simulink model "DynamicalMediationModel_Sim"  (R2015a)
settings: Solver=ode45  StartTime=0.0  StopTime=36  RelTol=1e-3
values from neighbouring files (symbols this model uses):
  out_model = pem(out_iddata',[pC_struct pB_struct])    [DynamicalModelingExercise_code.m]
  StepTime = 8    [DynamicalModelingExercise_code.m]
libraries: slident x3
settings Model: Creator=ktimms  LastModifiedBy=timmskep
settings DataIOCC: InitialState=ic_out_full  LimitDataPoints=off  SaveFormat=StructureWithTime  SignalLoggingSaveFormat=ModelDataLogs
settings OptimizationCC: ExpressionDepthLimit=2147483647
settings DebuggingCC: UnderspecifiedInitializationDetection=Classic  MergeDetectMultiDrivingBlocksExec=none  SolverPrmCheckMsg=warning  FcnCallInpInsideContextMsg=UseLocalSettings  StateNameClashWarn=warning
settings GRTTargetCC: CombineOutputUpdateFcns=off  GRTInterface=on

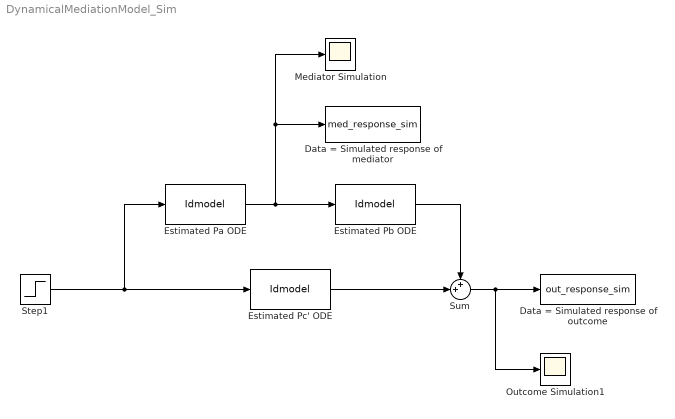
== system DynamicalMediationModel_Sim ==
  Data = Simulated response of mediator : ToWorkspace  VariableName=med_response_sim  SaveFormat=Structure With Time  SampleTime=1
  Data = Simulated response of outcome : ToWorkspace  VariableName=out_response_sim  SaveFormat=Structure With Time  SampleTime=1
  Estimated Pa ODE : slident/Models/Idmodel  sys=med_model  IC=0  noi=off  seed=[]
  Estimated Pb ODE : slident/Models/Idmodel  sys=out_model(2)  IC=0  noi=off  seed=[]
  Estimated Pc' ODE : slident/Models/Idmodel  sys=out_model(1)  IC=0  noi=off  seed=[]
  Mediator Simulation : Scope
      settings: YMin=-10  YMax=20  SaveName=ScopeData4
  Outcome Simulation1 : Scope
      settings: SaveName=ScopeData5
  Step1 : Step  Time=StepTime  SampleTime=0
  Sum : Sum  Inputs=++|
  wires:
  Estimated Pa ODE/1 -> Estimated Pb ODE/1, Mediator Simulation/1, Data = Simulated response of mediator/1
  Step1/1 -> Estimated Pc' ODE/1, Estimated Pa ODE/1
  Sum/1 -> Data = Simulated response of outcome/1, Outcome Simulation1/1
  Estimated Pb ODE/1 -> Sum/1
  Estimated Pc' ODE/1 -> Sum/2
